simulink model "testCartPendAlgConSim"  (R2024b)
settings: Solver=VariableStepAuto  StartTime=0.0  StopTime=40  RelTol=1e-3
InitFcn:
  | if (~exist('Xi_a', 'var'))
  |     testCartPendAlgCon;
  | end
  | 
  | % nominal parameters for actuator-augmented cart pendulum
  | M0 = 1.1;
  | m0 = 0.9;
  | g0 = 9.81;
  | L0 = 1;
  | cd0 = 1;
  | 
  | % backstepping controller parameters
  | a1 = 3;
  | a2 = 3;
  | a3 = 3;
  | a4 = 3;
  | 
  | % parameters for perturbed actuator-augmented cart pendulum
  | M = M0*1.0; % mass of cart [kg]
  | m = m0*2.0; % mass of pendulum [kg]
  | g = g0; % gravity acceleration [m/s^2]
  | L = L0; % length of pendulum [m]
  | cd = cd0; % pendulum damping coefficient [N*s/m]
  | 
  | % low-pass filter pole
  | b = -100;
  | 
  | % helper variables for perturbed cart pendulum
  | k1 = g/L;
  | k2 = cd/(m*L^2);
  | k3 = L*(M + m);
  | k4 = m*L;
  | k5 = m/(M + m);
StopFcn:
  | % extract time and output data
  | t = out.tout;
  | outs = out.outputs.signals.values;
  | 
  | % plot simulation output
  | figure
  | plot(t, outs, 'LineWidth', 2)
  | grid on
  | xlabel("t [s]")
  | ylabel("y_1 [rad]")
  | legend(["y_d", "y_{algcon}", "y_{backstep}"], 'location', 'best')
values from neighbouring files (symbols this model uses):
  psi_func = matlabFunction(psi, 'Vars', {x})    [NLS_vs_KoopmanCont.m]    (also in testCartPendAlgCon.m = matlabFunction(psi_CCK, 'Vars', {[p; x]}))
  Pss = ss(A, B, C, 0)    [testCartPendAlgCon.m]
  Xi_a = loops.Si*K    [testCartPendAlgCon.m]
settings Model: Creator=bkurkcu  LastModifiedBy=cphan

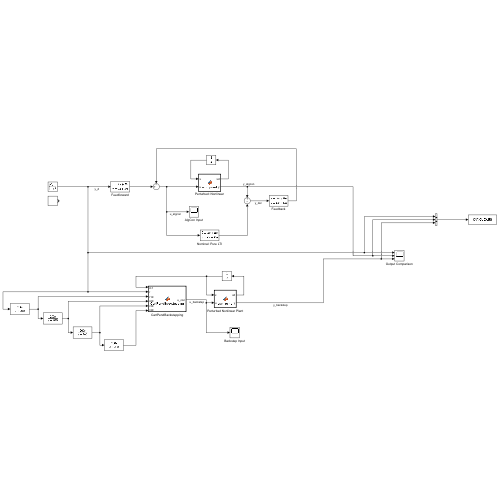
[thumbnail: Simulink's stored preview of the top-level diagram]
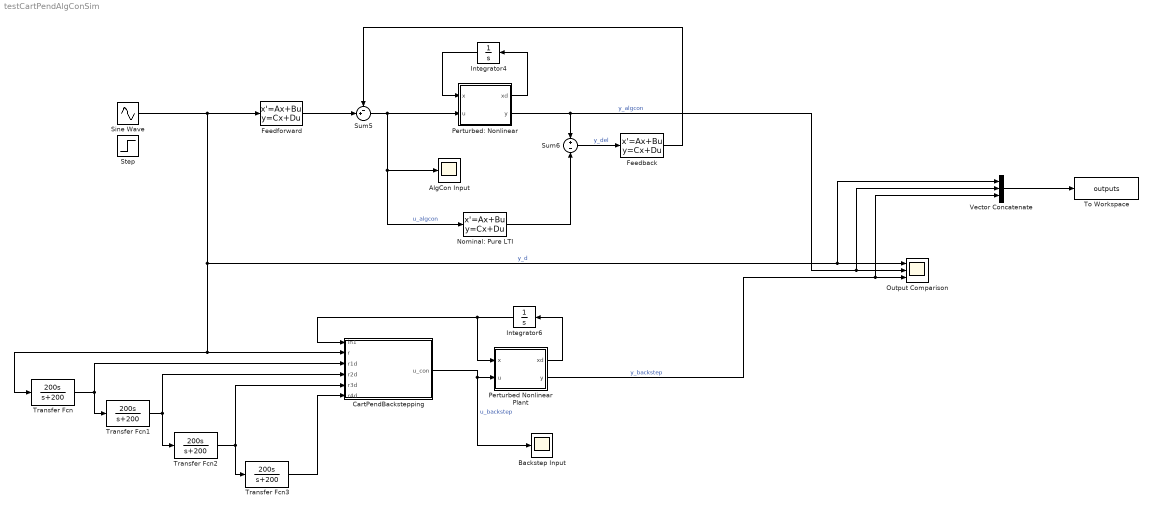
== system testCartPendAlgConSim ==
  AlgCon Input : Scope
  Backstep Input : Scope
  CartPendBackstepping : MATLAB Function  TreatAsAtomicUnit=on
  Feedback : StateSpace  A=Xi_a.a  B=Xi_a.b  C=Xi_a.c  D=Xi_a.d  InitialCondition=0
  Feedforward : StateSpace  A=Xi_a.a  B=Xi_a.b  C=Xi_a.c  D=Xi_a.d  InitialCondition=0
  Integrator4 : Integrator  InitialCondition=zeros(4, 1)
  Integrator6 : Integrator  InitialCondition=zeros(4, 1)
  Nominal: Pure LTI : StateSpace  A=Pss.a  B=Pss.b  C=Pss.c  D=Pss.d  InitialCondition=psi_func(zeros(4, 1))
  Output Comparison : Scope  NumInputPorts=3
  Perturbed Nonlinear Plant : MATLAB Function  TreatAsAtomicUnit=on
  Perturbed: Nonlinear : MATLAB Function  TreatAsAtomicUnit=on
  Sine Wave : Sin  Frequency=2*pi*0.05  SampleTime=0
  Step : Step  SampleTime=0
  Sum5 : Sum  Inputs=-+|
  Sum6 : Sum  Inputs=+|-
  To Workspace : ToWorkspace  VariableName=outputs  SaveFormat=Structure With Time  SampleTime=-1
  Transfer Fcn{,1..3} (4 alike) : TransferFcn  Numerator=[200 0]  Denominator=[1 200]
  Vector Concatenate : Concatenate  NumInputs=3
  wires:
  Nominal: Pure LTI/1 -> Sum6/2
  Sum5/1 -> Perturbed: Nonlinear/2(u), AlgCon Input/1, Nominal: Pure LTI/1  "u_algcon"
  Sum6/1 -> Feedback/1  "y_del"
  Feedforward/1 -> Sum5/2
  Perturbed: Nonlinear/2(y) -> Vector Concatenate/2, Output Comparison/2, Sum6/1  "y_algcon"
  Feedback/1 -> Sum5/1
  Integrator4/1 -> Perturbed: Nonlinear/1(x)
  Perturbed: Nonlinear/1(xd) -> Integrator4/1
  Integrator6/1 -> Perturbed Nonlinear Plant/1(x), CartPendBackstepping/1(in1)
  Perturbed Nonlinear Plant/1(xd) -> Integrator6/1
  CartPendBackstepping/1(u_con) -> Backstep Input/1, Perturbed Nonlinear Plant/2(u)  "u_backstep"
  Perturbed Nonlinear Plant/2(y) -> Vector Concatenate/3, Output Comparison/3  "y_backstep"
  Transfer Fcn/1 -> CartPendBackstepping/3(r1d), Transfer Fcn1/1
  Transfer Fcn1/1 -> CartPendBackstepping/4(r2d), Transfer Fcn2/1
  Transfer Fcn2/1 -> CartPendBackstepping/5(r3d), Transfer Fcn3/1
  Sine Wave/1 -> CartPendBackstepping/2(r), Transfer Fcn/1, Vector Concatenate/1, Output Comparison/1, Feedforward/1  "y_d"
  Transfer Fcn3/1 -> CartPendBackstepping/6(r4d)
  Vector Concatenate/1 -> To Workspace/1

== matlab function testCartPendAlgConSim/CartPendBackstepping ==
  data: in1 input; u_con output; r input; r1d input; r2d input; r3d input; r4d input; a1 parameter; a2 parameter; a3 parameter; a4 parameter
function u_con = CartPendBackstepping(in1,r,r1d,r2d,r3d,r4d,a1, a2, a3, a4)
%#codegen

%    This function was generated by the Symbolic Math Toolbox version 24.2.
%    17-Apr-2026 19:08:05

% in1 = complex(in1);  % if required to enforce complex operations
% r = complex(r);  % if required to enforce complex operations
% r1d = complex(r1d);  % if required to enforce complex operations
% r2d = complex(r2d);  % if required to enforce complex operations
% r3d = complex(r3d);  % if required to enforce complex operations
% r4d = complex(r4d);  % if required to enforce complex operations
% a1 = complex(a1);  % if required to enforce complex operations
% a2 = complex(a2);  % if required to enforce complex operations
% a3 = complex(a3);  % if required to enforce complex operations
% a4 = complex(a4);  % if required to enforce complex operations
p1 = in1(1,:);
p2 = in1(2,:);
x1 = in1(3,:);
x2 = in1(4,:);
t2 = cos(x1);
t3 = sin(x1);
t4 = a1.*a2;
t5 = x1.*2.0;
t6 = x2.^2;
t7 = x2.^3;
t16 = -x1;
t17 = -x2;
t24 = x2.*(1.0e+1./9.0);
t8 = cos(t5);
t9 = t2.^2;
t10 = t2.^3;
t12 = t2.^5;
t14 = sin(t5);
t15 = t3.^3;
t18 = p1.*t3.*5.0e+1;
t19 = t2.*9.81e+2;
t22 = (p1.*t2)./2.0;
t28 = t3.*(9.81e+2./1.0e+2);
t34 = t2.*t3.*t6.*(9.0./2.0e+1);
t11 = t9.^2;
t13 = t9.^3;
t20 = t8.*9.0;
t21 = t9.*9.0;
t23 = -t18;
t25 = t8.*8.1e+1;
t26 = t14.*x2.*1.62e+2;
t27 = t8.*(9.0./2.0);
t32 = t6.*t14.*(9.0./4.0e+1);
t42 = t22+t24+t28+t34;
t29 = t20-3.1e+1;
t30 = t21-2.0e+1;
t31 = t26+4.0e+2;
t33 = t25-2.79e+2;
t37 = t27-3.1e+1./2.0;
t43 = t22+t24+t28+t32;
t35 = 1.0./t30;
t38 = 1.0./t33;
t39 = 1.0./t37;
t36 = t35.^2;
t40 = t31.*t38;
t41 = a1+a2+t40;
et1 = a1.*3.6e+5+a3.*3.6e+5-t2.*3.1392e+6-t6.*9.0e+5+t10.*5.2974e+6-a1.*t2.*3.5316e+5-a2.*t2.*3.5316e+5-a3.*t2.*3.5316e+5+a1.*t6.*1.62e+5+a3.*t4.*3.6e+5+a2.*t6.*1.62e+5+a3.*t6.*1.62e+5-a1.*t9.*4.86e+5-a1.*t10.*1.430298e+6+a1.*t11.*2.187e+5-a2.*t10.*1.430298e+6-a3.*t9.*4.86e+5+a1.*t12.*7.15149e+5-a3.*t10.*1.430298e+6-a1.*t13.*3.2805e+4;
et2 = a2.*t12.*7.15149e+5+a3.*t11.*2.187e+5+a3.*t12.*7.15149e+5-a3.*t13.*3.2805e+4-p1.*t3.*4.7e+5+p2.*t3.*1.8e+5+p1.*t15.*2.7e+5+t6.*t9.*5.85e+5+t6.*t11.*8.1e+5-t7.*t14.*4.05e+4+t3.*x2.*7.663572e+6-t14.*x2.*4.0e+5-t15.*x2.*1.0488852e+7+a1.*p1.*t3.*1.8e+5+a2.*p1.*t3.*1.8e+5+a3.*p1.*t3.*1.8e+5-a1.*t6.*t9.*3.24e+5-a3.*t4.*t9.*4.86e+5-a2.*t6.*t9.*3.24e+5+a1.*t6.*t11.*1.12995e+5;
et3 = a3.*t4.*t11.*2.187e+5-a3.*t6.*t9.*3.24e+5+a2.*t6.*t11.*1.12995e+5-a3.*t4.*t13.*3.2805e+4+a3.*t6.*t11.*1.12995e+5+a1.*t14.*x2.*1.8e+5+a2.*t14.*x2.*1.8e+5+a3.*t14.*x2.*1.8e+5-p2.*t3.*t11.*3.645e+4-p1.*t2.*x2.*6.3e+5+p1.*t10.*x2.*7.533e+5+p1.*t12.*x2.*1.0935e+5+t3.*t7.*t10.*6.7797e+5+t3.*t11.*x2.*2.145447e+6-a1.*p1.*t3.*t11.*3.645e+4-a2.*p1.*t3.*t11.*3.645e+4-a3.*p1.*t3.*t11.*3.645e+4-a1.*t3.*t10.*x2.*1.62e+5;
et4 = a2.*t3.*t10.*x2.*-1.62e+5-a3.*t3.*t10.*x2.*1.62e+5;
et5 = r4d+r1d.*(a1+a3+a3.*t4)+r3d.*(a1+a2+a3)+a4.*(r1d+r3d+t17+a1.*(r+t16)+t17.*(t4+(t19+t23+t6.*t8.*4.5e+1)./(t8.*(4.5e+1./2.0)-1.55e+2./2.0)+t14.*t39.^2.*t43.*1.8e+2+1.0)+r1d.*(t4+1.0)+a3.*(r+r2d+t16+a1.*r1d+a1.*t17+a2.*(r1d+t17+a1.*r+a1.*t16)-(t3.*8.829e+3+x2.*1.0e+3+p1.*t2.*4.5e+2+t6.*t14.*(4.05e+2./2.0))./(t8.*(4.05e+2./2.0)-6.975e+2))+r2d.*(a1+a2)-p2.*t2.*t39.*1.0e+1-t39.*t41.*t43.*2.0e+1)+r2d.*(t4+a1.*a3+a2.*a3+2.0)+t2.*t35.*(p1.*1.0e+5+p2.*2.0e+3);
et6 = (t35.^3.*x2.*(et1+et2+et3+et4))./4.5e+1-t35.*t42.*(t4+a3.*t41-(t6.*4.5e+1+t18-t19-t6.*t9.*9.0e+1)./(t9.*4.5e+1-1.0e+2)+1.0./t29.^2.*x2.*(t14.*8.0e+2+x2.*3.24e+2-t8.*x2.*1.116e+3)+(t41.*(t14.*x2.*(9.0./2.0e+1)+1.0e+1./9.0).*4.0e+1)./t29+t2.*t3.*t36.*t42.*7.2e+2+2.0).*2.0e+1-p2.*t36.*(t2.*2.0e+2-a1.*t2.*1.8e+2-a2.*t2.*1.8e+2-a3.*t2.*1.8e+2+a1.*t10.*8.1e+1+a2.*t10.*8.1e+1+a3.*t10.*8.1e+1+t3.*x2.*1.8e+2+t3.*t9.*x2.*2.43e+2).*(1.0e+1./9.0);
u_con = ((et5+et6).*(t9.*(9.0./2.0e+1)-1.0))./(t2.*5.0e+3);
end

== matlab function testCartPendAlgConSim/Perturbed: Nonlinear ==
  data: x input; u input; xd output; k1 parameter; k2 parameter; k3 parameter; k4 parameter; k5 parameter; b parameter; y output
function [xd, y] = cart_pend(x, u, k1, k2, k3, k4, k5, b)

xd = [x(2);
      -b^2*x(1) + 2*b*x(2) + b^2*u;
      x(4);
      (-k1*sin(x(3)) - k2*x(4) - cos(x(3))/k3 .* (x(1) + k4*sin(x(3)).*x(4).^2))./(1 - k5*cos(x(3)).^2)];

y = x(3);

== matlab function testCartPendAlgConSim/Perturbed Nonlinear Plant ==
  data: x input; u input; xd output; k1 parameter; k2 parameter; k3 parameter; k4 parameter; k5 parameter; b parameter; y output
function [xd, y] = cart_pend(x, u, k1, k2, k3, k4, k5, b)

xd = [x(2);
      -b^2*x(1) + 2*b*x(2) + b^2*u;
      x(4);
      (-k1*sin(x(3)) - k2*x(4) - cos(x(3))/k3 .* (x(1) + k4*sin(x(3)).*x(4).^2))./(1 - k5*cos(x(3)).^2)];

y = x(3);
